simulink model "p_regulator"  (R2026a)
settings: Solver=VariableStepAuto  StopTime=2000
values from neighbouring files (symbols this model uses):
  K_mech = 1    [lab2.m]
  K_obj = 1    [lab2.m]
  K_p = 6    [lab2.m]
  K_sens = 3.9    [lab2.m]
  T1 = 100    [lab2.m]
  T2 = 250    [lab2.m]
  T_sens = 20    [lab2.m]
settings Model: Creator=Lenovo  LastModifiedBy=Lenovo

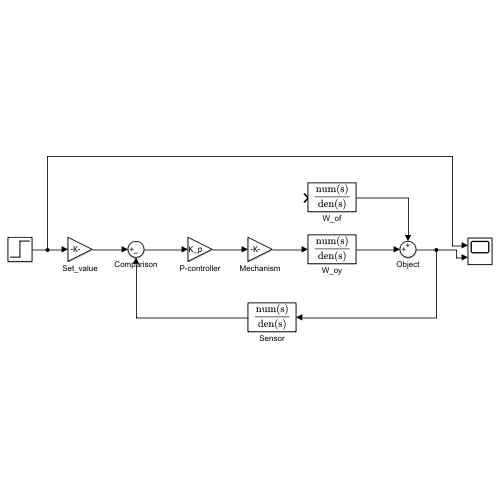
[thumbnail: Simulink's stored preview of the top-level diagram]
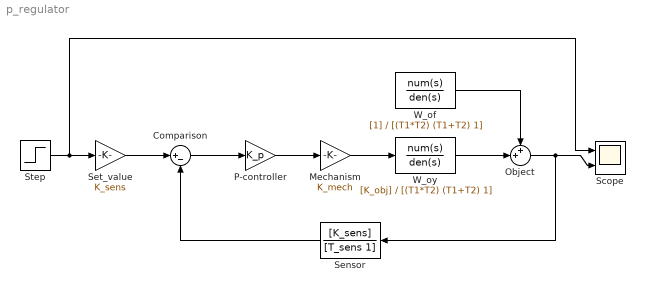
== system p_regulator ==
  Comparison : Sum  Inputs=|+-
  Mechanism : Gain  Gain=K_mech
  Object : Sum  Inputs=++|
  P-controller : Gain  Gain=K_p
  Scope : Scope  NumInputPorts=2
      settings: ActiveDisplayYMinimum=-0.12611547419634386  ActiveDisplayYMaximum=1.1350392677670951
  Sensor : TransferFcn  Numerator=[K_sens]  Denominator=[T_sens 1]
  Set_value : Gain  Gain=K_sens
  Step : Step  Time=0  SampleTime=0
  W_of : TransferFcn  Denominator=[(T1*T2) (T1+T2) 1]
  W_oy : TransferFcn  Numerator=[K_obj]  Denominator=[(T1*T2) (T1+T2) 1]
  wires:
  W_of/1 -> Object/1
  Mechanism/1 -> W_oy/1
  P-controller/1 -> Mechanism/1
  Comparison/1 -> P-controller/1
  Set_value/1 -> Comparison/1
  Sensor/1 -> Comparison/2
  Step/1 -> Set_value/1, Scope/1
  W_oy/1 -> Object/2
  Object/1 -> Sensor/1, Scope/2
